simulink model "LQG_UAV_LateralAP"  (R2019b)
settings: Solver=FixedStepAuto  StartTime=0.0  StopTime=20  FixedStep=0.005  RelTol=1e-3
values from neighbouring files (symbols this model uses):
  Ap_lat = [-0.000625746 0.00200502 -126.31 3.711;-0.149438 -1.74874 0.172113 0; 0.00783305 -0.085404 -0.001846 0; 0 1 0 0]    [LateralAP_FlightWing.m]
  Bp_lat = [-0.00370476 36.8612 -0.05977335 0]'    [LateralAP_FlightWing.m]
  Clo_lat = [0 1 0 0; 0 0 1 0; 0 0 0 1]    [LateralAP_FlightWing.m]
  Cp_lat = eye(4)    [LateralAP_FlightWing.m]
  Dp_lat = zeros(4,1)    [LateralAP_FlightWing.m]
  flag_act = flag_act_aux(i)    [runLQGSimulink.m]
  flag_controller = flag_controller_aux(i)    [runLQGSimulink.m]
  flag_noise = flag_noise_aux(i)    [runLQGSimulink.m]
  Klqg_lat = lqe(Ap_lat,eye(4),Clo_lat, Qf, Rn)    [LateralAP_FlightWing.m]
  Klqr_lat_gain = lqr(A_aug, B_aug, Q , R)    [LateralAP_FlightWing.m]
  wn_act = 5*2*pi    (= 31.4159265359)    [LateralAP_FlightWing.m]    (also in LonAP_FilghtWing.m)
  zeta_act = 0.7    [LateralAP_FlightWing.m]    (also in LonAP_FilghtWing.m)
undefined symbols (not defined in the file or in its folder): phi, prate, rrate, v
libraries: simulink x1
settings Model: Creator=adolf  LastModifiedBy=covasanvictor
settings DataIOCC: ReturnWorkspaceOutputs=off
settings DebuggingCC: ArithmeticOperatorsInVariantConditions=warning
settings SFSimCC: SimUseLocalCustomCode=off  CustomCodeUndefinedFunction=UseInterfaceOnly
settings RTWCC: RTWUseLocalCustomCode=off

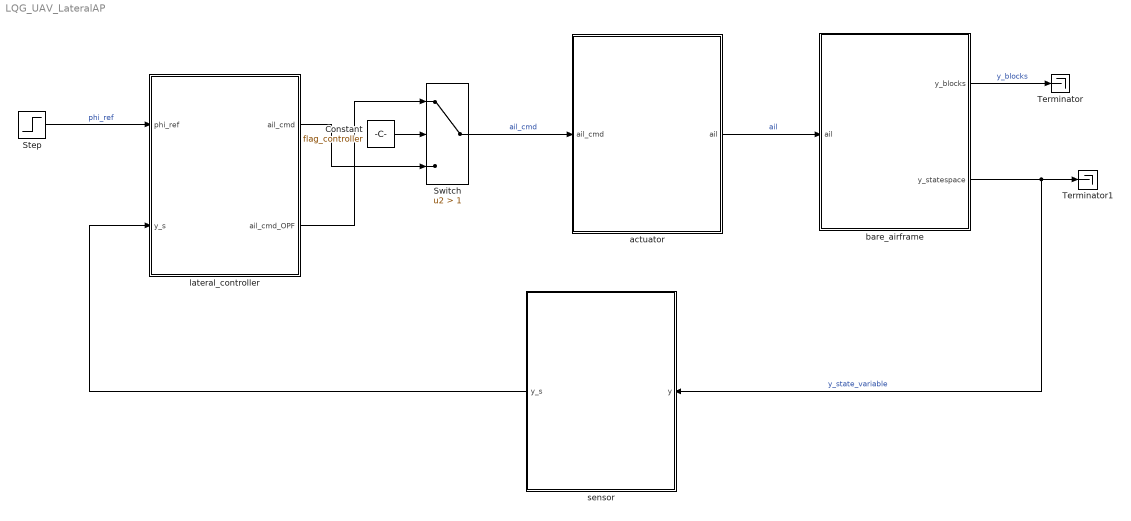
== system LQG_UAV_LateralAP ==
  Constant : Constant  Value=flag_controller
  Step : Step  SampleTime=0
  Switch : Switch  Criteria=u2 > Threshold  Threshold=1
  Terminator : Terminator
  Terminator1 : Terminator
  actuator : Subsystem
  bare_airframe : Subsystem
  lateral_controller : Subsystem
  sensor : Subsystem
  wires:
  bare_airframe/1(y_blocks) -> Terminator/1  "y_blocks"
  actuator/1(ail) -> bare_airframe/1(ail)  "ail"
  Step/1 -> lateral_controller/1(phi_ref)  "phi_ref"
  Constant/1 -> Switch/2
  lateral_controller/2(ail_cmd_OPF) -> Switch/1
  lateral_controller/1(ail_cmd) -> Switch/3
  Switch/1 -> actuator/1(ail_cmd)  "ail_cmd"
  sensor/1(y_s) -> lateral_controller/2("y_s ")
  bare_airframe/2(y_statespace) -> Terminator1/1, sensor/1(y)  "y_state_variable"

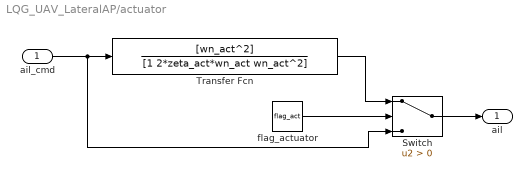
== system LQG_UAV_LateralAP/actuator ==
  ail_cmd : Inport
  Switch : Switch  Criteria=u2 > Threshold
  Transfer Fcn : TransferFcn  Numerator=[wn_act^2]  Denominator=[1 2*zeta_act*wn_act wn_act^2]
  flag_actuator : Constant  Value=flag_act
  ail : Outport  VectorParamsAs1DForOutWhenUnconnected=off
  wires:
  flag_actuator/1 -> Switch/2
  Switch/1 -> ail/1
  Transfer Fcn/1 -> Switch/1
  ail_cmd/1 -> Switch/3, Transfer Fcn/1

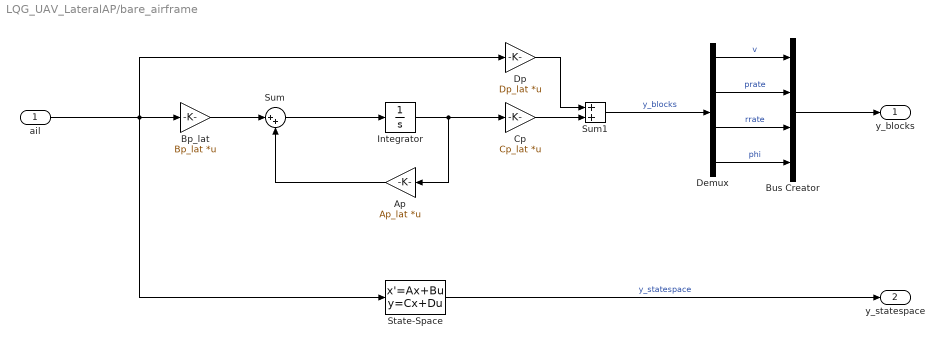
== system LQG_UAV_LateralAP/bare_airframe ==
  ail : Inport
  Ap : Gain  Gain=Ap_lat  Multiplication=Matrix(K*u) (u vector)
  Bp_lat : Gain  Gain=Bp_lat  Multiplication=Matrix(K*u) (u vector)
  Bus Creator : BusCreator  Inputs=v,prate,rrate,phi
  Cp : Gain  Gain=Cp_lat  Multiplication=Matrix(K*u) (u vector)
  Demux : Demux
  Dp : Gain  Gain=Dp_lat  Multiplication=Matrix(K*u) (u vector)
  Integrator : Integrator  InitialCondition=zeros(4,1)  ContinuousStateAttributes={'u', 'w','q','theta'}
  State-Space : StateSpace  A=Ap_lat  B=Bp_lat  C=Cp_lat  D=Dp_lat  InitialCondition=0
  Sum : Sum  Inputs=|++
  Sum1 : Sum
  y_blocks : Outport  VectorParamsAs1DForOutWhenUnconnected=off
  y_statespace : Outport  Port=2  VectorParamsAs1DForOutWhenUnconnected=off
  wires:
  State-Space/1 -> y_statespace/1  "y_statespace"
  Cp/1 -> Sum1/2
  Integrator/1 -> Ap/1, Cp/1
  Ap/1 -> Sum/2
  Bp_lat/1 -> Sum/1
  ail/1 -> State-Space/1, Dp/1, Bp_lat/1
  Dp/1 -> Sum1/1
  Sum/1 -> Integrator/1
  Sum1/1 -> Demux/1  "y_blocks"
  Demux/4 -> Bus Creator/4  "phi"
  Demux/3 -> Bus Creator/3  "rrate"
  Demux/2 -> Bus Creator/2  "prate"
  Demux/1 -> Bus Creator/1  "v"
  Bus Creator/1 -> y_blocks/1

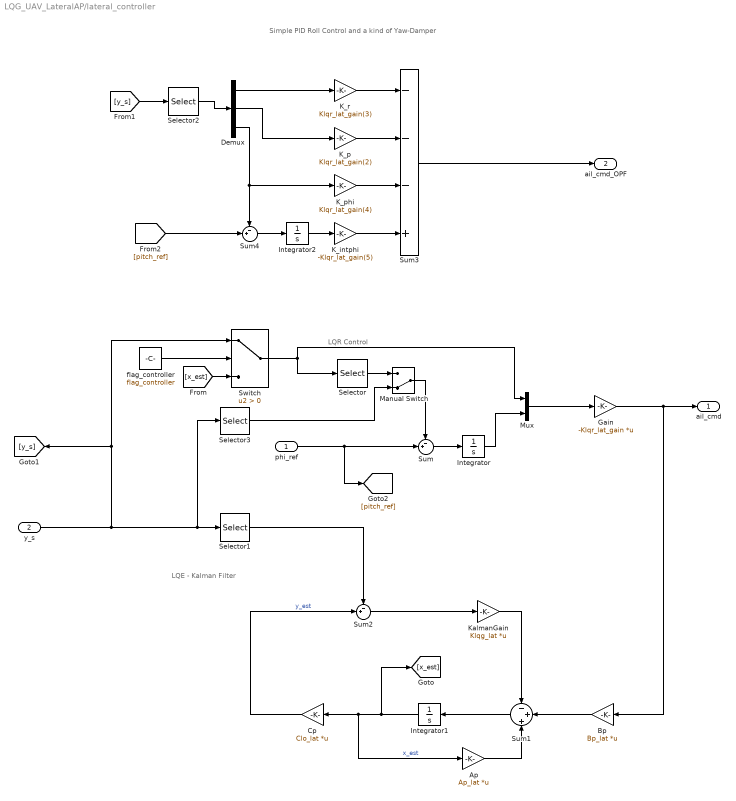
== system LQG_UAV_LateralAP/lateral_controller ==
  note: Simple PID Roll Control and a kind of Yaw-Damper
  note: LQR Control
  note: LQE - Kalman Filter
  phi_ref : Inport
  "y_s " : Inport  Port=2
  Ap : Gain  Gain=Ap_lat  Multiplication=Matrix(K*u) (u vector)
  Bp : Gain  Gain=Bp_lat  Multiplication=Matrix(K*u) (u vector)
  Cp : Gain  Gain=Clo_lat  Multiplication=Matrix(K*u) (u vector)
  Demux : Demux  Outputs=3
  Gain : Gain  Gain=-Klqr_lat_gain  Multiplication=Matrix(K*u) (u vector)
  Integrator : Integrator
  Integrator1 : Integrator  InitialCondition=zeros(4,1)  ContinuousStateAttributes={'v', 'p','r','phi'}
  Integrator2 : Integrator
  K_intphi : Gain  Gain=-Klqr_lat_gain(5)
  K_p : Gain  Gain=Klqr_lat_gain(2)
  K_phi : Gain  Gain=Klqr_lat_gain(4)
  K_r : Gain  Gain=Klqr_lat_gain(3)
  KalmanGain : Gain  Gain=Klqg_lat  Multiplication=Matrix(K*u) (u vector)
  Manual Switch : ManualSwitch  CurrentSetting=0
  Mux : Mux  Inputs=2
  Selector : Selector  InputPortWidth=4  IndexOptions=Index vector (dialog)  Indices=4  OutputSizes=1
  Selector1 : Selector  InputPortWidth=4  IndexOptions=Index vector (dialog)  Indices=[2 3 4]  OutputSizes=1
  Selector2 : Selector  InputPortWidth=4  IndexOptions=Index vector (dialog)  Indices=[3 2 4]  OutputSizes=1
  Selector3 : Selector  InputPortWidth=4  IndexOptions=Index vector (dialog)  Indices=4  OutputSizes=1
  Sum : Sum  Inputs=-+|
  Sum1 : Sum  Inputs=-++
  Sum2 : Sum  Inputs=-+|
  Sum3 : Sum  Inputs=---+
  Sum4 : Sum  Inputs=-+|
  Switch : Switch  Criteria=u2 > Threshold
  flag_controller : Constant  Value=flag_controller
  ail_cmd : Outport  VectorParamsAs1DForOutWhenUnconnected=off
  ail_cmd_OPF : Outport  Port=2  VectorParamsAs1DForOutWhenUnconnected=off
  wires:
  phi_ref/1 -> [pitch_ref], Sum/2
  Mux/1 -> Gain/1
  Sum/1 -> Integrator/1
  Integrator/1 -> Mux/2
  Gain/1 -> Bp/1, ail_cmd/1
  Sum1/1 -> Integrator1/1
  Integrator1/1 -> [x_est], Cp/1, Ap/1  "x_est"
  Ap/1 -> Sum1/3
  Bp/1 -> Sum1/2
  Cp/1 -> Sum2/2  "y_est"
  Selector1/1 -> Sum2/1
  Sum2/1 -> KalmanGain/1
  Switch/1 -> Selector/1, Mux/1
  flag_controller/1 -> Switch/2
  "y_s "/1 -> Switch/1, [y_s], Selector3/1, Selector1/1
  [x_est] -> Switch/3
  KalmanGain/1 -> Sum1/1
  Sum4/1 -> Integrator2/1
  Integrator2/1 -> K_intphi/1
  [y_s] -> Selector2/1
  Selector2/1 -> Demux/1
  [pitch_ref] -> Sum4/2
  Sum3/1 -> ail_cmd_OPF/1
  K_intphi/1 -> Sum3/4
  K_phi/1 -> Sum3/3
  K_p/1 -> Sum3/2
  K_r/1 -> Sum3/1
  Demux/1 -> K_r/1
  Demux/3 -> K_phi/1, Sum4/1
  Demux/2 -> K_p/1
  Selector3/1 -> Manual Switch/2
  Selector/1 -> Manual Switch/1
  Manual Switch/1 -> Sum/1

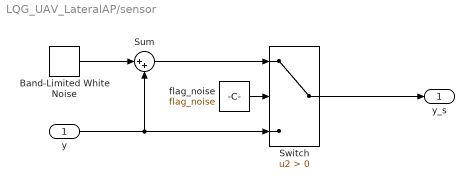
== system LQG_UAV_LateralAP/sensor ==
  y : Inport
  Band-Limited White Noise : simulink/Sources/Band-Limited White Noise  Cov=[0.0005 0.0005 0.0005 0.0001]  Ts=0.005  seed=[23341 23342 23343 23344]
  Sum : Sum  Inputs=|++
  Switch : Switch  Criteria=u2 > Threshold
  flag_noise : Constant  Value=flag_noise
  y_s : Outport  VectorParamsAs1DForOutWhenUnconnected=off
  wires:
  flag_noise/1 -> Switch/2
  Switch/1 -> y_s/1
  y/1 -> Sum/2, Switch/3
  Sum/1 -> Switch/1
  Band-Limited White Noise/1 -> Sum/1
